simulink model "Gleichstrommaschine_Validierung"  (R2022b)
settings: Solver=VariableStepAuto  StartTime=0.0  StopTime=10.0  RelTol=1e-3
settings Model: Creator=JSCHB  LastModifiedBy=JSCHB

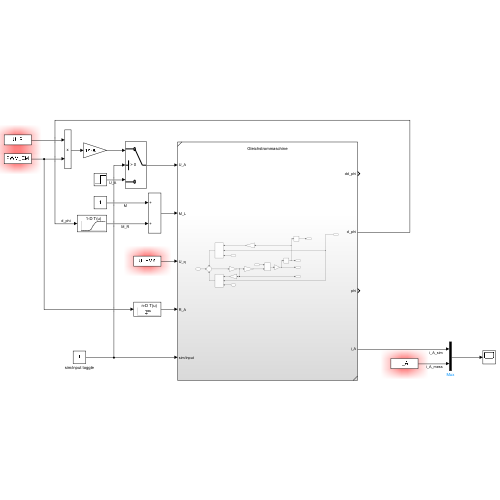
[thumbnail: Simulink's stored preview of the top-level diagram]
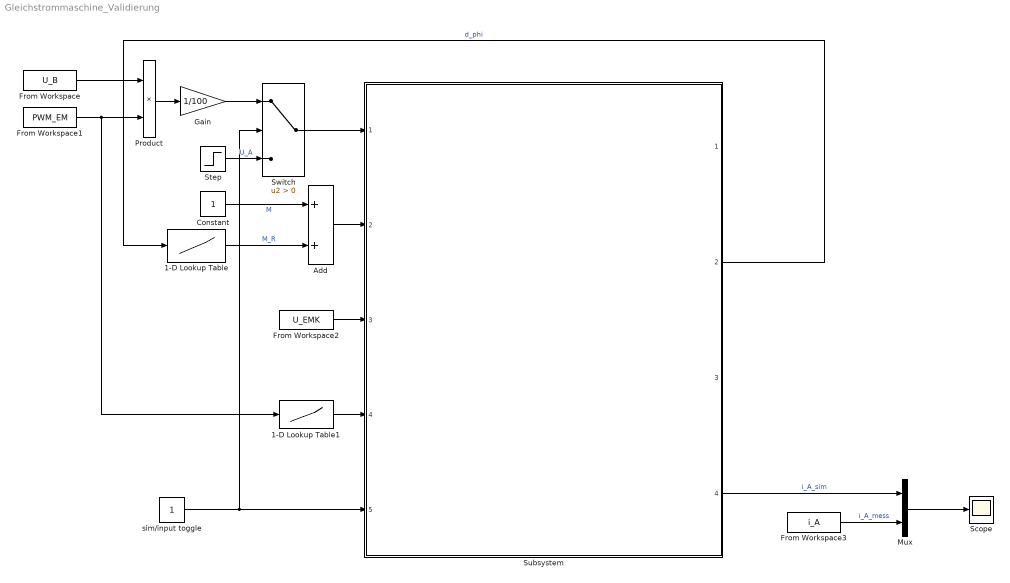
== system Gleichstrommaschine_Validierung ==
  1-D Lookup Table : Lookup_n-D  NumberOfTableDimensions=1  BreakpointsForDimension1=[-5:5]  Table=tanh([-5:5])  InternalRulePriority=Speed  RndMeth=Simplest
  1-D Lookup Table1 : Lookup_n-D  NumberOfTableDimensions=1  BreakpointsForDimension1="[0.57\t0.57\t0.2905\t0.2905\t0.255\t0.255\t0.207\t0.207]"  Table=[0.1 0.1 0.2 0.2 0.3 0.3 0.4 0.4]  InternalRulePriority=Speed  RndMeth=Simplest
  Add : Sum
  Constant : Constant
  From Workspace : FromWorkspace  VariableName=U_B
  From Workspace1 : FromWorkspace  VariableName=PWM_EM
  From Workspace2 : FromWorkspace  VariableName=U_EMK
  From Workspace3 : FromWorkspace  VariableName=i_A
  Gain : Gain  Gain=1/100
  Mux : Mux  Inputs=2
  Product : Product
  Scope : Scope
  Step : Step  SampleTime=0
  Subsystem : Subsystem  ReferencedSubsystem=Gleichstrommaschine
  Switch : Switch  Criteria=u2 > Threshold  SaturateOnIntegerOverflow=off  InputSameDT=off
  sim/input toggle : Constant
  wires:
  Constant/1 -> Add/1  "M"
  Add/1 -> Subsystem/2
  1-D Lookup Table/1 -> Add/2  "M_R"
  Subsystem/2 -> 1-D Lookup Table/1  "d_phi"
  From Workspace1/1 -> 1-D Lookup Table1/1, Product/2
  From Workspace/1 -> Product/1
  Product/1 -> Gain/1
  Switch/1 -> Subsystem/1
  Gain/1 -> Switch/1
  Step/1 -> Switch/3  "U_A"
  From Workspace2/1 -> Subsystem/3
  Subsystem/4 -> Mux/1  "i_A_sim"
  Mux/1 -> Scope/1
  From Workspace3/1 -> Mux/2  "i_A_mess"
  1-D Lookup Table1/1 -> Subsystem/4
  sim/input toggle/1 -> Switch/2, Subsystem/5
